simulink model "Equalizer"  (Simulink 8.7)
settings: Solver=ode45  StartTime=0.0  StopTime=inf  RelTol=1e-3
undefined symbols (not defined in the file or in its folder): gcbh, get, rcfiltgaincompat
libraries: commfilt2 x4, dspsnks4 x4, commrandsrc3 x1, commutil2 x1
settings Model: Creator=Administrator  LastModifiedBy=Administrator
settings DataIOCC: SignalLoggingSaveFormat=ModelDataLogs
settings OptimizationCC: ExpressionDepthLimit=2147483647  InitFltsAndDblsToZero=on
settings DebuggingCC: SaveWithParameterizedLinksMsg=none  SolverPrmCheckMsg=warning  FcnCallInpInsideContextMsg=UseLocalSettings  StateNameClashWarn=warning
settings GRTTargetCC: TargetFcnLib=ansi_tfl_tmw.mat  CombineOutputUpdateFcns=off  GRTInterface=on

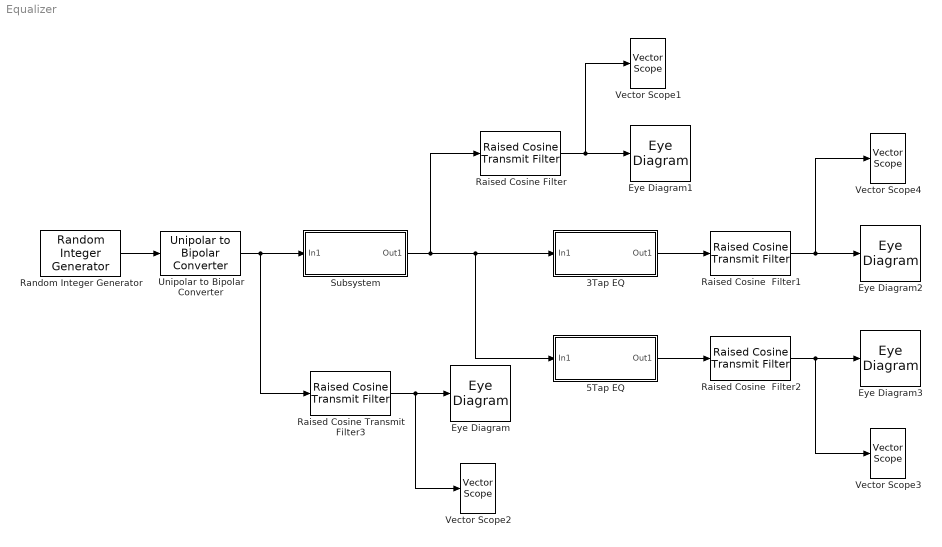
== system Equalizer ==
  3Tap EQ : Subsystem
  5Tap EQ : Subsystem
  Eye Diagram{,1..3} (4 alike) : EyeDiagram
  Raised Cosine  Filter1 : commfilt2/Raised Cosine Transmit Filter  filtType=Normal  R=1  filtSpan=2*(4)  N=8  filterGain=rcfiltgaincompat(gcbh)  InputProcessing=Columns as channels (frame based)  RateOptions=Enforce single-rate processing  framing=Mute  checkCoeff=off  variableName=rcTxFilt1  checkGain=Normalized  sampMode=Mute  saveAsFlag=0  currentFiltSpan=2*(4)  D=4  launchFVT=off  roundingMode=Floor  overflowMode=off  coeffDataTypeStr=Inherit: Same word length as input  coeffMin=[]  coeffMax=[]  coeffLastDataTypeStr=Inherit: Same word length as input  outputDataTypeStr=Inherit: Same as accumulator  outputMin=[]  outputMax=[]  outputLastDataTypeStr=Inherit: Same as accumulator
  Raised Cosine  Filter2 : commfilt2/Raised Cosine Transmit Filter  filtType=Normal  R=1  filtSpan=2*(4)  N=8  filterGain=rcfiltgaincompat(gcbh)  InputProcessing=Columns as channels (frame based)  RateOptions=Enforce single-rate processing  framing=Mute  checkCoeff=off  variableName=rcTxFilt2  checkGain=Normalized  sampMode=Mute  saveAsFlag=0  currentFiltSpan=2*(4)  D=4  launchFVT=off  roundingMode=Floor  overflowMode=off  coeffDataTypeStr=Inherit: Same word length as input  coeffMin=[]  coeffMax=[]  coeffLastDataTypeStr=Inherit: Same word length as input  outputDataTypeStr=Inherit: Same as accumulator  outputMin=[]  outputMax=[]  outputLastDataTypeStr=Inherit: Same as accumulator
  Raised Cosine Filter : commfilt2/Raised Cosine Transmit Filter  filtType=Normal  R=1  filtSpan=2*(4)  N=8  filterGain=rcfiltgaincompat(gcbh)  InputProcessing=Columns as channels (frame based)  RateOptions=Enforce single-rate processing  framing=Mute  checkCoeff=off  variableName=rcTxFilt  checkGain=Normalized  sampMode=Mute  saveAsFlag=0  currentFiltSpan=2*(4)  D=4  launchFVT=off  roundingMode=Floor  overflowMode=off  coeffDataTypeStr=Inherit: Same word length as input  coeffMin=[]  coeffMax=[]  coeffLastDataTypeStr=Inherit: Same word length as input  outputDataTypeStr=Inherit: Same as accumulator  outputMin=[]  outputMax=[]  outputLastDataTypeStr=Inherit: Same as accumulator
  Raised Cosine Transmit Filter3 : commfilt2/Raised Cosine Transmit Filter  filtType=Normal  R=1  filtSpan=2*(4)  N=8  filterGain=rcfiltgaincompat(gcbh)  InputProcessing=Columns as channels (frame based)  RateOptions=Enforce single-rate processing  framing=Mute  checkCoeff=off  variableName=rcTxFilt3  checkGain=Normalized  sampMode=Mute  saveAsFlag=0  currentFiltSpan=2*(4)  D=4  launchFVT=off  roundingMode=Floor  overflowMode=off  coeffDataTypeStr=Inherit: Same word length as input  coeffMin=[]  coeffMax=[]  coeffLastDataTypeStr=Inherit: Same word length as input  outputDataTypeStr=Inherit: Same as accumulator  outputMin=[]  outputMax=[]  outputLastDataTypeStr=Inherit: Same as accumulator
  Random Integer Generator : commrandsrc3/Random Integer Generator  SetSize=4  SeedSource=Parameter  Seed=37  SampleTime=1  SamplesPerFrame=1  OutputDataType=double  SimulateUsing=Interpreted execution
  Subsystem : Subsystem
  Unipolar to Bipolar Converter : commutil2/Unipolar to Bipolar Converter  M=4  polarity=Positive  dataType=Same as input
  Vector Scope{1..4} (4 alike) : dspsnks4/Vector Scope  ScopeProperties=on  Domain=Time  HorizSpan=10  DisplayProperties=off  AxisGrid=on  Memory=off  FrameNumber=on  AxisLegend=off  AxisZoom=off  OpenScopeAtSimStart=on  OpenScopeImmediately=off  FigPos=get(0,'defaultfigureposition')  AxisProperties=off  XUnits=Hertz  XRange=[0...Fs/2]  InheritXIncr=on  XIncr=1  XLabel=Time  XLimit=Auto  XMin=0  XMax=1  XStart=0  YUnits=dB  YLabel=Amplitude  LineProperties=off  XAxisParamsVer=6.8
      Vector Scope1 settings: YMin=-3.5  YMax=3.5
      Vector Scope2 settings: YMin=-3.32493815290218  YMax=3.31960750862153
      Vector Scope3 settings: YMin=-3.5  YMax=3.5
      Vector Scope4 settings: YMin=-3.2636439474748  YMax=3.01194035920016
  wires:
  Unipolar to Bipolar Converter/1 -> Subsystem/1(In1), Raised Cosine Transmit Filter3/1
  Subsystem/1(Out1) -> Raised Cosine Filter/1, 5Tap EQ/1(In1), 3Tap EQ/1(In1)
  Raised Cosine Filter/1 -> Eye Diagram1/1, Vector Scope1/1
  Raised Cosine  Filter1/1 -> Vector Scope4/1, Eye Diagram2/1
  Raised Cosine  Filter2/1 -> Eye Diagram3/1, Vector Scope3/1
  3Tap EQ/1(Out1) -> Raised Cosine  Filter1/1
  5Tap EQ/1(Out1) -> Raised Cosine  Filter2/1
  Raised Cosine Transmit Filter3/1 -> Eye Diagram/1, Vector Scope2/1
  Random Integer Generator/1 -> Unipolar to Bipolar Converter/1

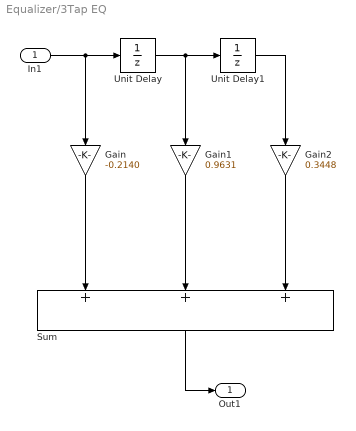
== system Equalizer/3Tap EQ ==
  In1 : Inport
  Gain : Gain  Gain=-0.2140
  Gain1 : Gain  Gain=0.9631
  Gain2 : Gain  Gain=0.3448
  Sum : Sum  Inputs=+++
  Unit Delay : UnitDelay
  Unit Delay1 : UnitDelay
  Out1 : Outport
  wires:
  Gain2/1 -> Sum/3
  Gain1/1 -> Sum/2
  Gain/1 -> Sum/1
  Unit Delay1/1 -> Gain2/1
  Unit Delay/1 -> Gain1/1, Unit Delay1/1
  In1/1 -> Gain/1, Unit Delay/1
  Sum/1 -> Out1/1

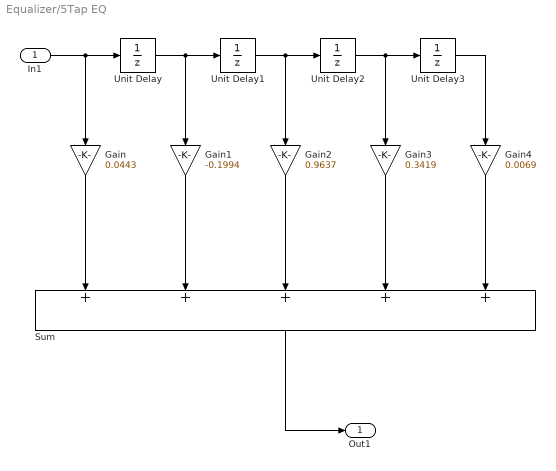
== system Equalizer/5Tap EQ ==
  In1 : Inport
  Gain : Gain  Gain=0.0443
  Gain1 : Gain  Gain=-0.1994
  Gain2 : Gain  Gain=0.9637
  Gain3 : Gain  Gain=0.3419
  Gain4 : Gain  Gain=0.0069
  Sum : Sum  Inputs=+++++
  Unit Delay{,1..3} (4 alike) : UnitDelay
  Out1 : Outport
  wires:
  In1/1 -> Unit Delay/1, Gain/1
  Unit Delay/1 -> Unit Delay1/1, Gain1/1
  Unit Delay1/1 -> Unit Delay2/1, Gain2/1
  Unit Delay2/1 -> Unit Delay3/1, Gain3/1
  Unit Delay3/1 -> Gain4/1
  Gain/1 -> Sum/1
  Gain1/1 -> Sum/2
  Gain2/1 -> Sum/3
  Gain3/1 -> Sum/4
  Gain4/1 -> Sum/5
  Sum/1 -> Out1/1

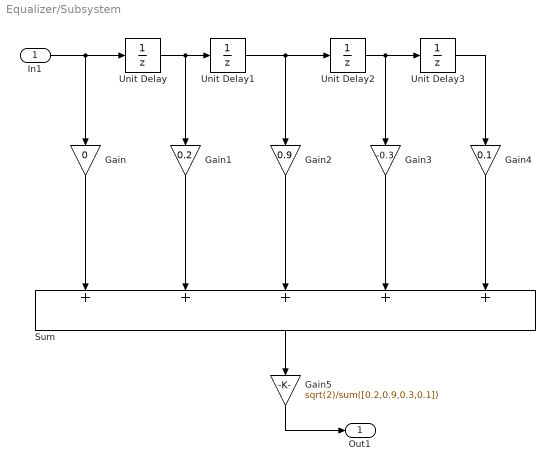
== system Equalizer/Subsystem ==
  In1 : Inport
  Gain : Gain  Gain=0
  Gain1 : Gain  Gain=0.2
  Gain2 : Gain  Gain=0.9
  Gain3 : Gain  Gain=-0.3
  Gain4 : Gain  Gain=0.1
  Gain5 : Gain  Gain=sqrt(2)/sum([0.2,0.9,0.3,0.1])
  Sum : Sum  Inputs=+++++
  Unit Delay{,1..3} (4 alike) : UnitDelay
  Out1 : Outport
  wires:
  In1/1 -> Unit Delay/1, Gain/1
  Unit Delay/1 -> Unit Delay1/1, Gain1/1
  Unit Delay1/1 -> Unit Delay2/1, Gain2/1
  Unit Delay2/1 -> Unit Delay3/1, Gain3/1
  Unit Delay3/1 -> Gain4/1
  Gain/1 -> Sum/1
  Gain1/1 -> Sum/2
  Gain2/1 -> Sum/3
  Gain3/1 -> Sum/4
  Gain4/1 -> Sum/5
  Sum/1 -> Gain5/1
  Gain5/1 -> Out1/1
